simulink model "Lab_1"  (R2021b)
settings: Solver=VariableStepAuto  StartTime=0.0  StopTime=1000  RelTol=1e-3
settings Model: Creator=ACL2022_14  LastModifiedBy=yjyoo

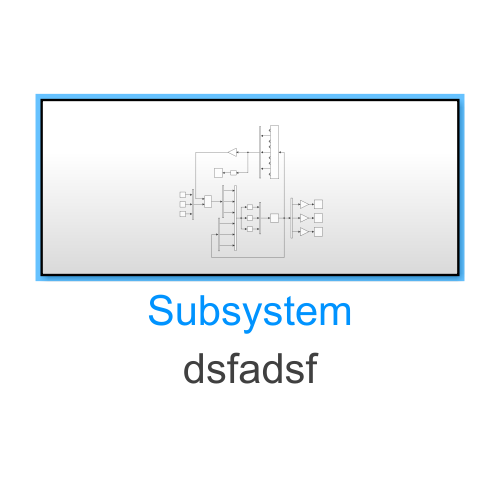
[thumbnail: Simulink's stored preview of the top-level diagram]
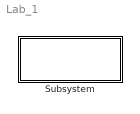
== system Lab_1 ==
  Subsystem : Subsystem
      settings: AttributesFormatString=dsfadsf

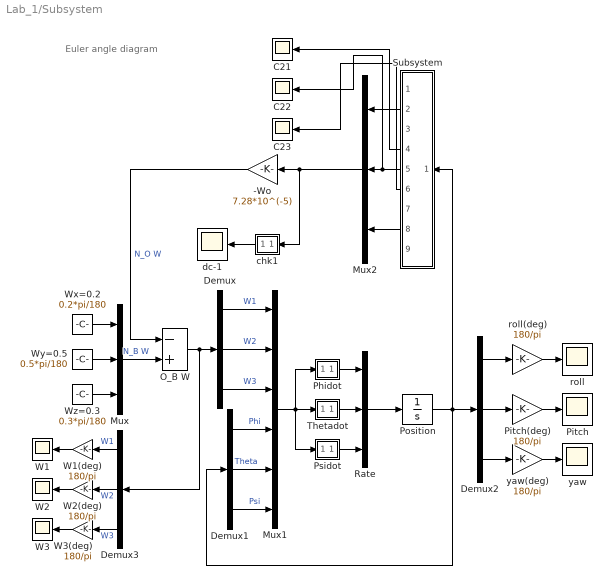
== system Lab_1/Subsystem ==
  note: Euler angle diagram
  -Wo : Gain  Gain=7.28*10^(-5)
  C21 : Scope
  C22 : Scope
  C23 : Scope
  Demux{,1..3} (4 alike) : Demux  Outputs=3
  Mux : Mux  Inputs=3
  Mux1 : Mux  Inputs=6
  Mux2 : Mux  Inputs=3
  O_B W : Sum  Inputs=-+
  Phidot : MATLAB Function  TreatAsAtomicUnit=on
  Pitch : Scope
  Pitch(deg) : Gain  Gain=180/pi
  Position : Integrator  InitialCondition=[10*pi/180, 20*pi/180, 30*pi/180]
  Psidot : MATLAB Function  TreatAsAtomicUnit=on
  Rate : Mux  Inputs=3
  Subsystem : Subsystem
  Thetadot : MATLAB Function  TreatAsAtomicUnit=on
  W1 : Scope
  W1(deg) : Gain  Gain=180/pi
  W2 : Scope
  W2(deg) : Gain  Gain=180/pi
  W3 : Scope
  W3(deg) : Gain  Gain=180/pi
  Wx=0.2 : Constant  Value=0.2*pi/180
  Wy=0.5 : Constant  Value=0.5*pi/180
  Wz=0.3 : Constant  Value=0.3*pi/180
  chk1 : MATLAB Function  TreatAsAtomicUnit=on
  dc-1 : Scope
  roll : Scope
  roll(deg) : Gain  Gain=180/pi
  yaw : Scope
  yaw(deg) : Gain  Gain=180/pi
  wires:
  Wy=0.5/1 -> Mux/2
  Wx=0.2/1 -> Mux/1
  Wz=0.3/1 -> Mux/3
  Mux/1 -> O_B W/2  "N_B W"
  -Wo/1 -> O_B W/1  "N_O W"
  O_B W/1 -> Demux3/1, Demux/1
  Mux1/1 -> Psidot/1(u), Phidot/1(u), Thetadot/1(u)
  Demux1/2 -> Mux1/5  "Theta"
  Demux/2 -> Mux1/2  "W2"
  Demux1/3 -> Mux1/6  "Psi"
  Demux/3 -> Mux1/3  "W3"
  Demux/1 -> Mux1/1  "W1"
  Phidot/1(y) -> Rate/1
  Thetadot/1(y) -> Rate/2
  Psidot/1(y) -> Rate/3
  Rate/1 -> Position/1
  Position/1 -> Subsystem/1(angle), Demux1/1, Demux2/1
  Demux2/1 -> roll(deg)/1
  Demux2/2 -> Pitch(deg)/1
  Demux2/3 -> yaw(deg)/1
  Pitch(deg)/1 -> Pitch/1
  roll(deg)/1 -> roll/1
  yaw(deg)/1 -> yaw/1
  Demux1/1 -> Mux1/4  "Phi"
  Subsystem/8(C32) -> Mux2/3
  Subsystem/5(C22) -> C22/1, Mux2/2
  Subsystem/2(C12) -> Mux2/1
  chk1/1(y) -> dc-1/1
  Mux2/1 -> chk1/1(u), -Wo/1
  Demux3/1 -> W1(deg)/1  "W1"
  Demux3/2 -> W2(deg)/1  "W2"
  Demux3/3 -> W3(deg)/1  "W3"
  W1(deg)/1 -> W1/1
  W2(deg)/1 -> W2/1
  W3(deg)/1 -> W3/1
  Subsystem/4(C21) -> C21/1
  Subsystem/6(C23) -> C23/1

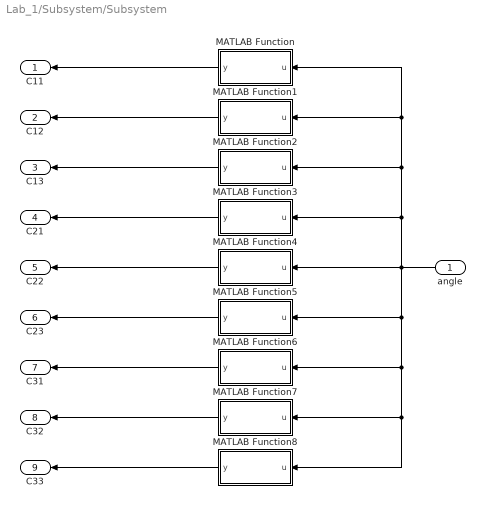
== system Lab_1/Subsystem/Subsystem ==
  angle : Inport
  MATLAB Function : MATLAB Function  TreatAsAtomicUnit=on
  MATLAB Function1 : MATLAB Function  TreatAsAtomicUnit=on
  MATLAB Function2 : MATLAB Function  TreatAsAtomicUnit=on
  MATLAB Function3 : MATLAB Function  TreatAsAtomicUnit=on
  MATLAB Function4 : MATLAB Function  TreatAsAtomicUnit=on
  MATLAB Function5 : MATLAB Function  TreatAsAtomicUnit=on
  MATLAB Function6 : MATLAB Function  TreatAsAtomicUnit=on
  MATLAB Function7 : MATLAB Function  TreatAsAtomicUnit=on
  MATLAB Function8 : MATLAB Function  TreatAsAtomicUnit=on
  C11 : Outport
  C12 : Outport  Port=2
  C13 : Outport  Port=3
  C21 : Outport  Port=4
  C22 : Outport  Port=5
  C23 : Outport  Port=6
  C31 : Outport  Port=7
  C32 : Outport  Port=8
  C33 : Outport  Port=9
  wires:
  angle/1 -> MATLAB Function8/1(u), MATLAB Function7/1(u), MATLAB Function6/1(u), MATLAB Function5/1(u), MATLAB Function4/1(u), MATLAB Function3/1(u), MATLAB Function2/1(u), MATLAB Function1/1(u), MATLAB Function/1(u)
  MATLAB Function/1(y) -> C11/1
  MATLAB Function1/1(y) -> C12/1
  MATLAB Function2/1(y) -> C13/1
  MATLAB Function3/1(y) -> C21/1
  MATLAB Function4/1(y) -> C22/1
  MATLAB Function5/1(y) -> C23/1
  MATLAB Function6/1(y) -> C31/1
  MATLAB Function7/1(y) -> C32/1
  MATLAB Function8/1(y) -> C33/1

== matlab function Lab_1/Subsystem/Phidot ==
  data: u input; y output
function y = Phidot(u)

y = u(1) + sin(u(4))*tan(u(5))*u(2) + cos(u(4))*tan(u(5))*u(3);

end

== matlab function Lab_1/Subsystem/Psidot ==
  data: u input; y output
function y = Psidot(u)

y = (sin(u(4))/cos(u(5)))*u(2) + (cos(u(4))/cos(u(5))*u(3));

end

== matlab function Lab_1/Subsystem/Subsystem/MATLAB Function ==
  data: u input; y output
function y = C11(u)

y = cos(u(3))*cos(u(2));

end

== matlab function Lab_1/Subsystem/Subsystem/MATLAB Function1 ==
  data: u input; y output
function y = C12(u)

y = sin(u(3))*cos(u(2));

end

== matlab function Lab_1/Subsystem/Subsystem/MATLAB Function2 ==
  data: u input; y output
function y = C13(u)

y = -sin(u(2));

end

== matlab function Lab_1/Subsystem/Subsystem/MATLAB Function3 ==
  data: u input; y output
function y = C21(u)

y = -sin(u(3))*cos(u(1)) + cos(u(3))*sin(u(2))*sin(u(1));

end

== matlab function Lab_1/Subsystem/Subsystem/MATLAB Function4 ==
  data: u input; y output
function y = C22(u)

y = cos(u(3))*cos(u(1)) + sin(u(3))*sin(u(2))*sin(u(1));

end

== matlab function Lab_1/Subsystem/Subsystem/MATLAB Function5 ==
  data: u input; y output
function y = C23(u)

y = cos(u(2))*sin(u(1));

end

== matlab function Lab_1/Subsystem/Thetadot ==
  data: u input; y output
function y = Thetadot(u)

y = cos(u(4))*u(2) - sin(u(4))*u(3);

end

== matlab function Lab_1/Subsystem/Subsystem/MATLAB Function6 ==
  data: u input; y output
function y = C31(u)

y = sin(u(3))*sin(u(1)) + cos(u(3))*sin(u(2))*cos(u(1));

end

== matlab function Lab_1/Subsystem/Subsystem/MATLAB Function7 ==
  data: u input; y output
function y = C32(u)

y = -cos(u(3))*sin(u(1)) + sin(u(3))*sin(u(2))*cos(u(1));

end

== matlab function Lab_1/Subsystem/Subsystem/MATLAB Function8 ==
  data: u input; y output
function y = C33(u)

y = cos(u(2))*cos(u(1));

end

== matlab function Lab_1/Subsystem/chk1 ==
  data: u input; y output
function y = chk1(u)

y = u(1)^2 + u(2)^2 + u(3)^2 - 1;

end
